simulink model "vertical_smm_with_lqr_3d"  (R2014b)
settings: Solver=FixedStepDiscrete  StartTime=0.0  StopTime=inf  FixedStep=sample_time  RelTol=1e-3
values from neighbouring files (symbols this model uses):
  forward_dx = [-0.304875592207 -0.274388032987 -0.243900473766 -0.213412914545 -0.182925355324 -0.152437796104 -0.121950236883 -0.0914626776622 -0.0609751184415 -0.0304875592207 0 0.0304875592207 ... (714 elements, 21x34)]    [ref_trajs.mat]
  forward_dx_of_dxstar = [-1.3048755994 -1.25487559904 -1.20487559868 -1.15487559832 -1.10487559796 -1.0548755976 -1.00487559724 -0.954875596883 -0.904875596523 -0.854875596164 -0.804875595804 -0.754875595707 ... (29274 elements, 41x21x34)]    [ref_trajs.mat]
  forward_x = [0.0961104217981 0.0864993796183 0.0768883374385 0.0672772952586 0.0576662530788 0.048055210899 0.0384441687192 0.0288331265394 0.0192220843596 0.00961104217981 0 -0.00961104217981 ... (714 elements, 21x34)]    [ref_trajs.mat]
  forward_x_of_dxstar = [0.247353819189 0.239791649319 0.232229479449 0.22466730958 0.21710513971 0.209542969841 0.201980799971 0.194418630102 0.186856460232 0.179294290363 0.171732120493 0.164169950675 ... (29274 elements, 41x21x34)]    [ref_trajs.mat]
  target_dx_range = [-1 -0.95 -0.9 -0.85 -0.8 -0.75 -0.7 -0.65 -0.6 -0.55 -0.5 -0.45 ... (41 elements, 1x41)]    [ref_trajs.mat]
undefined symbols (not defined in the file or in its folder): A_kalman_fourbar_gear, A_kalman_transverse, A_kalman_vertical, A_lpf_dtau, A_lpf_leg_spring, B1_lpf_dtau, B1_lpf_leg_spring, B2_lpf_dtau, B2_lpf_leg_spring, B_dx_versus_x0, B_kalman_fourbar_gear, B_kalman_transverse, B_kalman_vertical, backwards_K_front_of_t_row1, backwards_K_front_of_t_row2, backwards_K_sag_of_t, C_kalman_fourbar_gear, C_kalman_transverse, C_kalman_vertical, com_leg_motor, com_torso, contact_threshold, control_start_time, d_vertical_com, deadbeat_enabled, desired_com_forward_velocity, desired_com_lateral_velocity, desired_initial_leg_roll_left, desired_initial_leg_roll_right, desired_lateral_symmetry_angle, desired_torso_pitch, desired_torso_roll, Discrete, fcut_contact, forward_velocity_target_step, g, HIP_MTR_MAX_CONT_TORQUE, i_leg_motor, i_robot, i_torso, initial_dx_estimate, initial_dy_estimate, initial_dz_estimate, initial_z_estimate, j_motor, j_segments, K_left_lat_flight, K_left_lat_flight_winch, k_LQR_vertical, K_right_lat_flight, K_right_lat_flight_winch, k_sea, k_vertical_winch, kalman_load_to_deflect_transmission, kalman_stance_slip_threshold, kd_motor, kp_motor, l_retract_delta, l_retract_swing_max, l_retract_swing_min ... (+58)
libraries: simulink x8, ctrlSharedLib x7
(part 4 of 4)

== matlab function vertical_smm_with_lqr_3d/Control/Behavior Control/Primary Leg Behavior/Running/Stance/COM X,Y,Z  trajectory generation ==
  data: enable_hopping input; x_0 output size=1; y_0 output size=1; z_ref output size=1; dz_ref output size=1; ddz_ref output size=1; x_ref output size=1; dx_ref output size=1; y_ref output size=1; dy_ref output size=1; t input size=1; dx0 input; dy0 input; target_DX input; target_DY input; z_rest_new parameter; z_amplitude parameter; spring_frequency parameter; phase_0 parameter; forward_x_of_dxstar parameter; forward_dx_of_dxstar parameter; forward_x parameter; forward_dx parameter; target_dx_range parameter; T_s parameter
%% COM trajectory generation for stance & foot placement for flight

% Outputs:
% x_0: desired x position for foot at touchdown
% y_0: desired y position for foot at touchdown
% [z_ref, dz_ref, ddz_ref]: reference trajectory for vertical
% [x_ref, dx_ref]: reference trajectory for forward
% [y_ref, dy_ref]: reference trajectory for lateral

% Inputs:
% t: time since touchdown
% dx0: touchdown x velocity
% dy0: touchdown y velocity
% target_DX: desired x velocity at takeoff
% s_duration: nominal stance time
% z_rest_new: z height of oscillation
% target_dx_range: full range of possible x velocities in lookup table
% forward_x_of_dxstar: master lookup table for x trajectories
% T_s: tabled vector from 0 to s_duration

function [x_0, y_0,...
          z_ref, dz_ref, ddz_ref, ...
          x_ref, dx_ref, y_ref, dy_ref] ...
          = ReferenceTrajectory(enable_hopping, t, dx0, dy0, target_DX, target_DY, z_rest_new, z_amplitude, ...
            spring_frequency, phase_0, forward_x_of_dxstar, forward_dx_of_dxstar, ...
            forward_x, forward_dx, target_dx_range, T_s)
        
  % Z trajectory during stance
    if enable_hopping
        z_ref =  z_rest_new + z_amplitude*sin(spring_frequency*t+phase_0);
        dz_ref = z_amplitude*spring_frequency*cos(spring_frequency*t+phase_0);
        ddz_ref = -z_amplitude*spring_frequency^2*sin(spring_frequency*t+phase_0);
    else
        z_ref = z_rest_new - z_amplitude;
        dz_ref = 0;
        ddz_ref = 0;
    end
    
  % [X, dX] trajectory from 0 to s_duration
  forward_x_given_dxstar = squeeze(interp1(target_dx_range, forward_x_of_dxstar, target_DX));
  forward_dx_given_dxstar = squeeze(interp1(target_dx_range, forward_dx_of_dxstar, target_DX));
    
  % saturate t and initial velocity to reference library
  t_sat = max( min(t, T_s(end)), 0);
  dx0 = max( min(dx0, max(forward_dx_given_dxstar(:,1))), min(forward_dx_given_dxstar(:,1)) );
  x_ref  = interp2(T_s, forward_dx_given_dxstar(:,1), forward_x_given_dxstar, t_sat, dx0);
  dx_ref = interp2(T_s, forward_dx_given_dxstar(:,1), forward_dx_given_dxstar, t_sat, dx0);
  x_0 = interp1(forward_dx_given_dxstar(:,1), forward_x_given_dxstar(:,1), dx0);

  % for now, keep dy_star = 0;
  dy0 = max( min(dy0, max(forward_dx(:,1))), min(forward_dx(:,1)) );
  y_ref =  interp2(T_s, forward_dx(:,1), forward_x, t_sat, dy0);
  dy_ref = interp2(T_s, forward_dx(:,1), forward_dx, t_sat, dy0);
  y_0 = interp1(forward_dx(:,1), forward_x(:,1), dy0);
end

== matlab function vertical_smm_with_lqr_3d/Control/Behavior Control/Primary Leg Behavior/Running/Stance/Lookup finite horizon LQR gain ==
  data: K_sag output; t_forward input; backwards_K_sag_of_t parameter; backwards_K_front_of_t_row1 parameter; backwards_K_front_of_t_row2 parameter; T_lqr parameter; stance_duration parameter; K_front output
%% Interpolates pregenerated finite horizon LQR gain tables 
% sagittal_state: [X, Pitch, dX, dPtich]
% frontal state: [Y; Roll; sym; dY; dRoll; angular_momentum];
function [K_sag, K_front]  =  FiniteHorizonLQRLookup(t_forward, backwards_K_sag_of_t, backwards_K_front_of_t_row1, backwards_K_front_of_t_row2, T_lqr, stance_duration)
  t = stance_duration - t_forward; % gains are scheduled w.r.t time until end.                                     
  t = min(max(t, min(T_lqr)), max(T_lqr));
  K_sag = interp1(T_lqr, backwards_K_sag_of_t, t);

  % inputs for frontal LQR: backwards_K_front_of_t_row1, backwards_K_front_of_t_row2
  K_front_row1 = interp1(T_lqr, backwards_K_front_of_t_row1, t);
  K_front_row2 = interp1(T_lqr, backwards_K_front_of_t_row2, t);
  K_front = [K_front_row1; K_front_row2];
end

== matlab function vertical_smm_with_lqr_3d/Control/Behavior Control/Primary Leg Behavior/Running/Flight/Convert Foot Position to Joint Angles + Leg Length  ==
  data: deadbeat input; desired_leg_length output; X_star input; Y_star input; Z_star input; right_left input; com_pelvis_body input; desired_alpha output; desired_beta output; dcom_pelvis_body input; roll input; pitch input; sagittal_angle input; lateral_angle input; leg_length input; lateral_offset parameter; max_leg_length parameter; desired_initial_leg_roll_right parameter; desired_initial_leg_roll_left parameter; z_land parameter; d_vertical_com parameter
function [ desired_leg_length, desired_alpha, desired_beta ]  =  ...
          ConvertToJointAnglesAndLegLength(deadbeat, X_star, Y_star, Z_star, right_left,...
                           com_pelvis_body, dcom_pelvis_body, ...
                           roll, pitch, sagittal_angle, lateral_angle, leg_length,...
                           lateral_offset, max_leg_length, desired_initial_leg_roll_right, desired_initial_leg_roll_left, z_land, d_vertical_com) 

    q = [roll(1), pitch(1), sagittal_angle(1), lateral_angle(1), leg_length(1)];
    dq = [roll(2), pitch(2), sagittal_angle(2), lateral_angle(2), leg_length(2)];
    [desired_alpha, desired_beta, desired_leg_length]  =  ConvertFootPositionToLegAnglesAndLegLength(X_star, Y_star, Z_star, right_left, com_pelvis_body, dcom_pelvis_body, q, dq, lateral_offset, max_leg_length);   
                       
    if ~deadbeat
        desired_leg_length = [z_land-d_vertical_com; 0; 0];
        desired_alpha = [pi; 0; 0];
        desired_beta = [desired_initial_leg_roll_left; 0; 0];
        if right_left
            desired_beta = [desired_initial_leg_roll_right; 0; 0];
        end
    end
    
end

== matlab function vertical_smm_with_lqr_3d/Control/Behavior Control/Primary Leg Behavior/Running/Circular Buffer/Buffer7 ==
  data: data input; buffer output size=recorded_steps; trigger input; buffer_size input
function buffer  = buffer_data(data, trigger, buffer_size)

    persistent buffer_memory
    coder.varsize('buffer_memory',100);
    if isempty(buffer_memory)
        buffer_memory = [];
    end
    
    if trigger
        buffer_memory = [data; buffer_memory];
        if size(buffer_memory, 1) > buffer_size
            buffer_memory = buffer_memory(1:buffer_size,:);
        end
    end
    
    buffer = buffer_memory;

end

== matlab function vertical_smm_with_lqr_3d/Control/Behavior Control/Secondary Leg Behavior/Virtual Leg to Four Bar ==
  data: l_leg input; dl_leg input; ddl_leg input; phi input; dphi input; ddphi input; back output; dback output; ddback output; front output; dfront output; ddfront output
function [back, dback, ddback, front, dfront, ddfront] = VirtualLegToFourBar(l_leg, dl_leg, ddl_leg, phi, dphi, ddphi)
    [back, dback, ddback, front, dfront, ddfront] = VirtualLegToFourBar(l_leg, dl_leg, ddl_leg, phi, dphi, ddphi);
end

== matlab function vertical_smm_with_lqr_3d/Control/Behavior Control/Primary Leg Behavior/Running/Closed Loop Compensation/CLOSED LOOP COMPENSATION X FOR VAIRABLE SPEED ==
  data: A_cl input; epsilon input; c input; delta_s_i input; dx_star input; B_cl input; delta_ux output
function delta_ux  = closed_loop_compensation_dxstar...
         (A_cl,epsilon, c, delta_s_i, dx_star, B_cl)
% assume form of delta_s_{i+1} = A_cl*delta_s_i + epsilon +c*dx_star + B_cl*delta_ux
% where delta measures deviation from deadbeat case. solve for
% delta_ux = (-A_cl*delta_s_i-epsilon - c*dxstar)/B_cl to achieve deadbeat
delta_ux = (-A_cl*delta_s_i - epsilon - c*dx_star)/B_cl;

== matlab function vertical_smm_with_lqr_3d/Control/Behavior Control/Primary Leg Behavior/Running/Closed Loop Compensation/ESTIMATE CLOSED LOOP ERROR X FOR VARIABLE SPEED ==
  data: dx_land_hist input; A_cl output; delta_ux_hist input; dx_lift_hist input; dx_star_hist input; B_dx_versus_x0 parameter; W_real input; epsilon_0 output; c output; A_cl_nb output; epsilon_0_nb output; c_nb output
function [A_cl, epsilon_0, c, ...
          A_cl_nb, epsilon_0_nb, c_nb] = error_fitting_dxstar...
         (dx_land_hist, delta_ux_hist, dx_lift_hist, dx_star_hist,...
          B_dx_versus_x0, W_real)
% data_length = min([length(dx_lift_hist), filter_length]);
data_length = length(dx_lift_hist);
assert(data_length < 100);
% add fake data
fake_dx_land_err_magnitude = 0.1; fake_dx_star_magnitude = 0.1;
[fgrid_dx_land_err, fgrid_dx_star, fgrid_dx_lift_err] = ...
    meshgrid(fake_dx_land_err_magnitude*[-1 1],fake_dx_star_magnitude*[-1 1],0);
fake_data_length = numel(fgrid_dx_land_err);
fake_dx_land_err = fgrid_dx_land_err(:);
fake_dx_star = fgrid_dx_star(:);
fake_dx_lift_err = fgrid_dx_lift_err(:);
fake_delta_ux = zeros(fake_data_length,1);
% assert(fake_data_length<100);
% assert(filter_length<100);
% fake_dx_land_err = linspace(-0.1, 0.1, fake_data_length)';
% fake_dx_lift_err = zeros(fake_data_length,1);
% fake_delta_ux = zeros(fake_data_length,1);
% fake_dx_star = linspace(-0.25, 0.25, fake_data_length)';
dx_land_err = [reshape(dx_land_hist(1:data_length)-dx_star_hist(1:data_length),...
                       data_length, 1); fake_dx_land_err];
dx_lift_err = [reshape(dx_lift_hist(1:data_length)-dx_star_hist(1:data_length),...
                       data_length, 1); fake_dx_lift_err];
dx_star = [reshape(dx_star_hist(1:data_length), data_length,1); fake_dx_star];
delta_ux = [reshape(delta_ux_hist(1:data_length), data_length, 1); fake_delta_ux];
% weighted least squares
W = diag([W_real*ones(1,data_length), ones(1,fake_data_length)]);
Y = dx_lift_err - B_dx_versus_x0*delta_ux;
X = [dx_land_err, dx_star, ones(data_length+fake_data_length,1)];
% linear regression for s_{i+1}-s0 = A_cl*(s_i-s0) + epsilon_0 + c(s0) + B*delta_u
% solve for Y = X*beta, beta column vector
beta_hat = (X'*W*X)\X'*W*Y;
W_nobias = diag([W_real*ones(1,data_length), 0.001*ones(1,fake_data_length)]);
beta_hat_nobias = (X'*W_nobias*X)\X'*W_nobias*Y;
A_cl = beta_hat(1);
c = beta_hat(2);
epsilon_0 = beta_hat(3);
A_cl_nb = beta_hat_nobias(1);
c_nb = beta_hat_nobias(2);
epsilon_0_nb = beta_hat_nobias(3);

== matlab function vertical_smm_with_lqr_3d/Control/Behavior Control/Primary Leg Behavior/Running/Closed Loop Compensation/CLOSED LOOP COMPENSATION Y FOR VAIRABLE SPEED ==
  data: A_cl input; epsilon input; c input; delta_s_i input; dx_star input; B_cl input; delta_ux output
function delta_ux  = closed_loop_compensation_dxstar...
         (A_cl,epsilon, c, delta_s_i, dx_star, B_cl)
% assume form of delta_s_{i+1} = A_cl*delta_s_i + epsilon +c*dx_star + B_cl*delta_ux
% where delta measures deviation from deadbeat case. solve for
% delta_ux = (-A_cl*delta_s_i-epsilon - c*dxstar)/B_cl to achieve deadbeat
delta_ux = (-A_cl*delta_s_i - epsilon - c*dx_star)/B_cl;

== matlab function vertical_smm_with_lqr_3d/Control/Behavior Control/Primary Secondary Leg Swap/ToggleRightLeftLeg ==
  data: toggle input boolean; right_left output double; previous_right_left input double
function right_left = ToggleRightLeftLeg(toggle, previous_right_left)
    
    if toggle
        right_left = -previous_right_left + 1;
    else
        right_left = previous_right_left;
    end

end

== matlab function vertical_smm_with_lqr_3d/Control/Behavior Control/Force Estimation/3D Forward Dynamics yawed ==
  data: right_or_left input; torso_roll input size=2; torso_pitch input double size=2; torso_yaw input double size=2; primary_sagittal_leg_angle input double size=2; primary_leg_length input double size=2; primary_leg_roll input double size=2; secondary_leg_roll input double size=2; primary_leg_torque input; primary_leg_force input; primary_lateral_torque input; secondary_lateral_torque input; R_GRF output double size=3; L_GRF output size=3; ddroll output double; g parameter; m_leg_motor parameter; m_torso parameter; i_torso parameter; i_leg_motor parameter; lateral_offset parameter; com_torso parameter
%% Forward 3D ATRIAS dynamics
function [R_GRF, L_GRF, ddroll]  =  ForwardDynamics3D(right_or_left, ...
                                                      torso_roll, torso_pitch, torso_yaw, ...
                                                      primary_sagittal_leg_angle, primary_leg_length,...
                                                      primary_leg_roll, secondary_leg_roll, ...
                                                      primary_leg_torque, primary_leg_force, ...
                                                      primary_lateral_torque, secondary_lateral_torque, ...
                                                      g, m_leg_motor, m_torso, i_torso, i_leg_motor, lateral_offset, com_torso)

    d = norm(com_torso(2:3));
    It = mean(i_torso);
    Im = mean(i_leg_motor);
    
    phi    = torso_roll(1);                    % roll
    theta  = torso_pitch(1);                   % pitch
    alpha1 = primary_sagittal_leg_angle(1);    % primary sagittal leg angle
    beta1  = primary_leg_roll(1);              % primary leg roll
    beta2  = secondary_leg_roll(1);            % secondary leg roll
    l1     = primary_leg_length(1);            % primary leg length
    
    dphi    = torso_roll(2);
    dtheta  = torso_pitch(2);
    dpsi    = torso_yaw(2);
    dalpha1 = primary_sagittal_leg_angle(2);
    dbeta1  = primary_leg_roll(2);
    dbeta2  = secondary_leg_roll(2);
    dl1     = primary_leg_length(2);
    
    
    tau_a1 = primary_leg_torque;
    tau_b1 = primary_lateral_torque;
    tau_b2 = secondary_lateral_torque;
    F_l1 = primary_leg_force;

    if right_or_left == 1
      A = A_fwd_yawed_right(lateral_offset,d,m_leg_motor,m_torso,It,Im,phi,theta,alpha1,beta1,beta2,l1);
      B = B_fwd_yawed_right(lateral_offset,d,g,m_leg_motor,m_torso,It,Im,phi,theta,alpha1,beta1,beta2,l1,dphi,dtheta,dpsi,dalpha1,dbeta1,dbeta2,dl1,tau_a1,tau_b1,tau_b2,F_l1);
    else
      A = A_fwd_yawed_left(lateral_offset,d,m_leg_motor,m_torso,It,Im,phi,theta,alpha1,beta1,beta2,l1);
      B = B_fwd_yawed_left(lateral_offset,d,g,m_leg_motor,m_torso,It,Im,phi,theta,alpha1,beta1,beta2,l1,dphi,dtheta,dpsi,dalpha1,dbeta1,dbeta2,dl1,tau_a1,tau_b1,tau_b2,F_l1);
    end
    
    x_fwd = A \ B;
    ddroll = x_fwd(4);
    GRF = zeros(3,1);
    GRF(1) = x_fwd(11);
    GRF(2) = x_fwd(12);
    GRF(3) = x_fwd(13); 
    
    if right_or_left == 1
        R_GRF = GRF;
        L_GRF = [0;0;0];
    else
        R_GRF = [0;0;0];
        L_GRF = GRF;
    end
end

== matlab function vertical_smm_with_lqr_3d/Control/Behavior Control/Primary Leg Behavior/Running/Flight/Avoid Hitting Mechanical Limits ==
  data: back_cmd output double; front_cmd output double; dback_cmd output double; dfront_cmd output double; ddback_cmd output double; ddfront_cmd output double; back_desired input; dback_desired input; ddback_desired input; front_desired input; dfront_desired input; ddfront_desired input; min_front_bar_angle parameter; max_front_bar_angle parameter; min_back_bar_angle parameter; max_back_bar_angle parameter
%% Avoid joint limits by ensuring we don't command velocities/accelerations that would push us into them when we are close to them.
function [back_cmd, front_cmd, dback_cmd, dfront_cmd, ddback_cmd, ddfront_cmd] ...
    = AvoidFourbarLimits(back_desired,dback_desired, ddback_desired, ...
          front_desired, dfront_desired, ddfront_desired, ...
          min_front_bar_angle, max_front_bar_angle, min_back_bar_angle, max_back_bar_angle)
    [back_cmd, front_cmd, dback_cmd, dfront_cmd, ddback_cmd, ddfront_cmd] = AvoidFourbarLimits(back_desired,dback_desired, ddback_desired, front_desired, dfront_desired, ddfront_desired, min_front_bar_angle, max_front_bar_angle, min_back_bar_angle, max_back_bar_angle);
end

== matlab function vertical_smm_with_lqr_3d/Control/Behavior Control/Primary Leg Behavior/Running/Flight/Virtual Leg to Four Bar ==
  data: l_leg input; dl_leg input; ddl_leg input; phi input; dphi input; ddphi input; back output; dback output; ddback output; front output; dfront output; ddfront output
function [back, dback, ddback, front, dfront, ddfront] = VirtualLegToFourBar(l_leg, dl_leg, ddl_leg, phi, dphi, ddphi)
    [back, dback, ddback, front, dfront, ddfront] = VirtualLegToFourBar(l_leg, dl_leg, ddl_leg, phi, dphi, ddphi);
end

== matlab function vertical_smm_with_lqr_3d/Control/Behavior Control/Primary Leg Behavior/Running/Flight/Lateral Flight Control ==
  data: hopping input; tau_primary output; tau_secondary output; RightLeftPrimary input; TorsoRoll input; LLegRoll input; RLegRoll input; Beta1_star input; Roll_star input; K_right_lat_flight parameter; K_left_lat_flight parameter; K_right_lat_flight_winch parameter; K_left_lat_flight_winch parameter; Q_phibeta1beta2 parameter; Q_phibeta1beta2_winch parameter; m_torso parameter; m_leg_motor parameter; com_torso parameter; i_torso parameter; i_leg_motor parameter; g parameter; lateral_offset parameter; adjusted_ref output; feedforward output; desired_initial_leg_roll_left parameter; desired_initial_leg_roll_right parameter
% full_state = [Roll; Beta1; Beta2; dRoll; dBeta1; dBeta2];
function [tau_primary, tau_secondary, ...
          adjusted_ref, feedforward] = lateral_flight_control(hopping, RightLeftPrimary,...
          TorsoRoll, LLegRoll, RLegRoll, Beta1_star, Roll_star,...
          K_right_lat_flight, K_left_lat_flight, K_right_lat_flight_winch, K_left_lat_flight_winch, Q_phibeta1beta2, Q_phibeta1beta2_winch,...
          m_torso, m_leg_motor, com_torso, i_torso, i_leg_motor, g, lateral_offset, desired_initial_leg_roll_left, desired_initial_leg_roll_right)

    d = norm(com_torso(2:3));
    It_f = i_torso(1);
    Im_f = i_leg_motor(1); 
    phidphi = TorsoRoll; 
    symdsym = LLegRoll-RLegRoll;
    ang_mom = phidphi(2)*(m_torso*d^2 + It_f + 2*(m_leg_motor*lateral_offset^2+ Im_f)) -symdsym(2)*(m_leg_motor*lateral_offset^2+Im_f);

    if RightLeftPrimary == 1
        Beta1 = RLegRoll;
        Beta2 = LLegRoll;
        Beta2_star = [desired_initial_leg_roll_left; 0; 0];
    else
        Beta1 = LLegRoll;
        Beta2 = RLegRoll;
        Beta2_star = [desired_initial_leg_roll_right; 0; 0];
    end    
    
    if ~hopping
        Q_phibeta1beta2 = Q_phibeta1beta2_winch;
        K_right_lat_flight = K_right_lat_flight_winch;
        K_left_lat_flight = K_left_lat_flight_winch;
    end

    ref_old = [Roll_star(1); Beta1_star(1); Beta2_star(1)];
    dref_old = [0; Beta1_star(2); Beta2_star(2)];
    ddref_old = [0; Beta1_star(3); Beta2_star(3)];
    
    % eliminate beta2 from state using momentum:
    % s_old = T*s_new+D(t); s_new = [phi; beta1];
    % dbeta_R = L/(Im_f+mm*r^2) - (It_f+mm*d^2+2*Im_f+2*mm*r^2)/(Im_f+mm*r^2)*dphi + dbeta_L 
    % beta_R = beta_R0 + L/(Im_f+mm*r^2)*t - ((It_f+mm*d^2+2*Im_f+2*mm*r^2)/(Im_f+mm*r^2)*(phi-phi0) + (beta_L-beta_L0)
    % beta_R = [beta_R0-b1*phi0-b2*beta_L0 + a*t + b1*phi + b2*beta_L;
    
    if RightLeftPrimary == 1 % beta_2 is beta_L, beta_1 is beta_R, eliminate beta2
      a = -ang_mom/(Im_f+m_leg_motor*lateral_offset^2);
      b1 = (It_f+m_torso*d^2+2*Im_f+2*m_leg_motor*lateral_offset^2)/(Im_f+m_leg_motor*lateral_offset^2); b2 = 1;
    else
      a = +ang_mom/(Im_f+m_leg_motor*lateral_offset^2);
      b1 = -(It_f+m_torso*d^2+2*Im_f+2*m_leg_motor*lateral_offset^2)/(Im_f+m_leg_motor*lateral_offset^2); b2 = 1;
    end
    
    T = [eye(2); b1, b2];
    %  D = [0; 0; 0; 0; beta_R0 - b1*phi0 - b2*beta_L0 + a*t; a];
    D = [0;0; Beta2(1) - b1*phidphi(1) - b2*Beta1(1)];
    
    % old cost (state s)  (s-s_ref)' * Q *(s-s_ref);
    % new cost (state r) =(T*r+D-s_ref)'*Q*(T*r+D-s_ref);
    %                    =(r+ (T'QT)^{-1}T'Q(D-s_ref))'*T'QT*
    %                     (r + (T'QT)^{-1}T'Q(D-s_ref))
    
    
    Q_new = T'*Q_phibeta1beta2*T;
    ref_new = Q_new\T'*Q_phibeta1beta2*(ref_old-D);
    ref_new_vel = Q_new\T'*Q_phibeta1beta2*(dref_old - [0;0; a]);
    ref_accels = Q_new\T'*Q_phibeta1beta2*(ddref_old);

    % A_phidphi_betadbeta1 = [0 1 0 0; 0 0 0 0; 0 0 0 1; 0 0 0 0];
    % assume beta1 is right
    if RightLeftPrimary == 1
        B_new_state = [0 0; 0 0; -1/(It_f+m_torso*d^2), 1/(It_f+m_torso*d^2); 1/(It_f+m_torso*d^2)+1/(Im_f+m_leg_motor*lateral_offset^2), -1/(It_f+m_torso*d^2)];
    else
        B_new_state = [0 0; 0 0; 1/(It_f+m_torso*d^2), -1/(It_f+m_torso*d^2); 1/(It_f+m_torso*d^2)+1/(Im_f+m_leg_motor*lateral_offset^2), -1/(It_f+m_torso*d^2)];
    end      
    
    %   K = lqr(A_phidphi_betadbeta1, B_phidphi_betadbeta1, Q_new, R_lat_flight);
    if RightLeftPrimary == 1
      K = K_right_lat_flight;
    else
      K = K_left_lat_flight;
    end

    new_state = [phidphi(1); Beta1(1); phidphi(2); Beta1(2)];
    new_ref_traj = [ref_new; ref_new_vel];

    feedforward = B_new_state([3 4],:)\ref_accels;
    if ~hopping, feedforward = -(m_leg_motor)*g*lateral_offset*ones(2,1); end
    tau_lqr = feedforward - K*(new_state-new_ref_traj);
    tau_1 = tau_lqr(1); tau_2 = tau_lqr(2);
    implied_beta2_star = [0 0 1]*(T*ref_new+D);
    implied_dbeta2_star = [0 0 1]*(T*ref_new_vel+[0; 0; a]);
    % implied_betadbeta2_star = [0 0 0 0 1 0; 0 0 0 0 0 1]*(T*ref_new+D);
    adjusted_ref = [ref_new; implied_beta2_star; ref_new_vel; implied_dbeta2_star];

    tau_primary = tau_1;
    tau_secondary = tau_2;

== matlab function vertical_smm_with_lqr_3d/Control/Behavior Control/Secondary Leg Behavior/Mirrored Leg Length Target ==
  data: primary_l_leg input; l_leg output; dl_leg output; primary_dl_leg input; l_retract_swing_min parameter; l_retract_swing_max parameter; ddl_leg output; l_retract_delta parameter
function [l_leg, dl_leg, ddl_leg] = LegLengthTarget(primary_l_leg, primary_dl_leg, l_retract_swing_min, l_retract_swing_max, l_retract_delta)

    l_leg = primary_l_leg - l_retract_delta;
    dl_leg = 0;
    ddl_leg = 0;
    if l_leg > l_retract_swing_min && l_leg < l_retract_swing_max
        dl_leg = primary_dl_leg;
    else
        l_leg = max(min(l_leg, l_retract_swing_max), l_retract_swing_min);
    end

end

== matlab function vertical_smm_with_lqr_3d/Fourbar Gearside Kalman Filter/External Trunk Torque Estimate ==
  data: grf_xz input; rotor_torque input; spring_torque input; tau_trunk output; torso_pitch input; d_vertical_com parameter; LEG_MTR_GEAR_RATIO parameter
function tau_trunk = tau_trunk(grf_xz, rotor_torque, spring_torque, torso_pitch, d_vertical_com, LEG_MTR_GEAR_RATIO )
    d = d_vertical_com;
    theta = torso_pitch;
    N = LEG_MTR_GEAR_RATIO;
    tau_trunk = sum(-rotor_torque + -(N-1)/N*spring_torque) + (-d*cos(theta)*grf_xz(1) + d*sin(theta)*grf_xz(2));
end

== matlab function vertical_smm_with_lqr_3d/Fourbar Gearside Kalman Filter/Covariance Estimates ==
  data: spring_torque input; absolute_gear input; current_position_estimate input; state_uncertainty input; Q1 output; R1 output; Q2 output; R2 output; R_kalman_absolute_normal parameter; R_kalman_absolute_fail parameter; R_kalman_incremental_unloaded parameter; R_kalman_incremental_loaded parameter; kalman_load_to_deflect_transmission parameter; Q3 output; R3 output; Q4 output; R4 output; max_absolute_measurement_innovation parameter; k_sea parameter; Q_kalman_spring_torque parameter; Q_kalman_rotor_torque parameter; Q_kalman_trunk_torque parameter; sample_time parameter
function [Q1, R1, Q2, R2, Q3, R3, Q4, R4] = covariance( spring_torque, absolute_gear, current_position_estimate, state_uncertainty, R_kalman_absolute_normal, R_kalman_absolute_fail, R_kalman_incremental_unloaded, R_kalman_incremental_loaded, kalman_load_to_deflect_transmission, max_absolute_measurement_innovation, k_sea, Q_kalman_spring_torque, Q_kalman_rotor_torque, Q_kalman_trunk_torque, sample_time)

    persistent previous_absolute_gear
    if isempty(previous_absolute_gear)
        previous_absolute_gear = absolute_gear;
    end
    
    % Measurement covariance
    R_absolute = ones(4,1)*R_kalman_absolute_normal;
    dropped_out = previous_absolute_gear == absolute_gear;
    out_of_range = abs(current_position_estimate - absolute_gear) > max_absolute_measurement_innovation;
    R_absolute(dropped_out | out_of_range) = R_kalman_absolute_fail;
    
    R_incremental_scale = min(abs(spring_torque)/kalman_load_to_deflect_transmission, 1);
    R_incremental = R_incremental_scale*R_kalman_incremental_loaded + (1-R_incremental_scale)*R_kalman_incremental_unloaded;
    
    R1 = diag([R_absolute(1), R_incremental(1)])/sample_time;
    R2 = diag([R_absolute(2), R_incremental(2)])/sample_time;
    R3 = diag([R_absolute(3), R_incremental(3)])/sample_time;
    R4 = diag([R_absolute(4), R_incremental(4)])/sample_time;
    
    % Process noise covariance
    Q_spring_torque = k_sea'.^2.*(state_uncertainty + R_kalman_absolute_normal) + Q_kalman_spring_torque;

    Q1 = diag([Q_spring_torque(1), Q_kalman_rotor_torque, Q_kalman_trunk_torque]);
    Q2 = diag([Q_spring_torque(2), Q_kalman_rotor_torque, Q_kalman_trunk_torque]);
    Q3 = diag([Q_spring_torque(3), Q_kalman_rotor_torque, Q_kalman_trunk_torque]);
    Q4 = diag([Q_spring_torque(4), Q_kalman_rotor_torque, Q_kalman_trunk_torque]);

    previous_absolute_gear = absolute_gear;
end

== matlab function vertical_smm_with_lqr_3d/Fourbar Gearside Kalman Filter/eigen values 1 ==
  data: Z input; E output
function E = eigen(Z)
    E = real(eig(Z));
    E = sort(E);
end

== matlab function vertical_smm_with_lqr_3d/Fourbar Gearside Kalman Filter/eigen values 2 ==
  data: Z input; E output
function E = eigen(Z)
    E = real(eig(Z));
    E = sort(E);
end

== matlab function vertical_smm_with_lqr_3d/Fourbar Gearside Kalman Filter/eigen values 3 ==
  data: Z input; E output
function E = eigen(Z)
    E = real(eig(Z));
    E = sort(E);
end

== matlab function vertical_smm_with_lqr_3d/Fourbar Gearside Kalman Filter/eigen values4  ==
  data: Z input; E output
function E = eigen(Z)
    E = real(eig(Z));
    E = sort(E);
end

== matlab function vertical_smm_with_lqr_3d/Control/Behavior Control/Primary Leg Behavior/Running/Stance/3D Inverse Dynamics yawed ==
  data: right_or_left input; primary_leg_torque output double size=1; torso_roll input double size=2; torso_pitch input double size=2; torso_yaw input size=2; primary_sagittal_leg_angle input size=2; primary_leg_length input size=2; primary_leg_roll input size=2; secondary_leg_roll input size=2; GRF_desired input double size=3; ddRoll_desired input double size=1; g parameter; primary_lateral_torque output double size=1; secondary_lateral_torque output double size=1; primary_leg_force output double size=1; m_leg_motor parameter; m_torso parameter; i_torso parameter; i_leg_motor parameter; lateral_offset parameter; com_torso parameter
%% Inverse dynamics
function [primary_leg_torque, primary_lateral_torque, secondary_lateral_torque, primary_leg_force]  =  InverseDynamics3D(right_or_left,...
                                                                                                                         torso_roll, torso_pitch, torso_yaw, ...
                                                                                                                         primary_sagittal_leg_angle, primary_leg_length, ...
                                                                                                                         primary_leg_roll, secondary_leg_roll, ...
                                                                                                                         GRF_desired, ddRoll_desired, ...
                                                                                                                         g, m_leg_motor, m_torso, i_torso, i_leg_motor, lateral_offset, com_torso)

    d = norm(com_torso(2:3));
    It = mean(i_torso);
    Im = mean(i_leg_motor);
    
    phi    = torso_roll(1);                    % roll
    theta  = torso_pitch(1);                   % pitch
    alpha1 = primary_sagittal_leg_angle(1);    % primary sagittal leg angle
    beta1  = primary_leg_roll(1);              % primary leg roll
    beta2  = secondary_leg_roll(1);            % secondary leg roll
    l1     = primary_leg_length(1);            % primary leg length
    
    dphi    = torso_roll(2);
    dtheta  = torso_pitch(2);
    dpsi    = torso_yaw(2);
    dalpha1 = primary_sagittal_leg_angle(2);
    dbeta1  = primary_leg_roll(2);
    dbeta2  = secondary_leg_roll(2);
    dl1     = primary_leg_length(2);

    Fx = GRF_desired(1);
    Fy = GRF_desired(2);
    Fz = GRF_desired(3);
    ddphi = ddRoll_desired;

    if right_or_left == 1
      A = A_id_roll_yawed_right(lateral_offset,d,m_leg_motor,m_torso,It,Im,phi,theta,alpha1,beta1,beta2,l1);     
      B = B_id_roll_yawed_right(lateral_offset,d,g,m_leg_motor,m_torso,It,Im,phi,theta,alpha1,beta1,beta2,l1,dphi,dtheta,dpsi,dalpha1,dbeta1,dbeta2,dl1,Fx,Fy,Fz,ddphi);
    else
      A = A_id_roll_yawed_left(lateral_offset,d,m_leg_motor,m_torso,It,Im,phi,theta,alpha1,beta1,beta2,l1);     
      B = B_id_roll_yawed_left(lateral_offset,d,g,m_leg_motor,m_torso,It,Im,phi,theta,alpha1,beta1,beta2,l1,dphi,dtheta,dpsi,dalpha1,dbeta1,dbeta2,dl1,Fx,Fy,Fz,ddphi);
    end        
    x_id_roll = A \ B;
    primary_leg_torque = x_id_roll(10);
    primary_lateral_torque = x_id_roll(11);
    secondary_lateral_torque = x_id_roll(12);
    primary_leg_force = x_id_roll(13);
end

== matlab function vertical_smm_with_lqr_3d/Control/Behavior Control/Primary Leg Behavior/Running/Flight/Avoid Virtual Leg Length Limits ==
  data: l_leg_desired input; dl_leg_desired input; ddl_leg_desired input; l_leg_cmd output double; dl_leg_cmd output double; ddl_leg_cmd output double; min_leg_length parameter; max_leg_length parameter
%% Avoid virtual leg length limits by ensuring we don't command position/velocities/accelerations that would hit them.
function [l_leg_cmd, dl_leg_cmd, ddl_leg_cmd] = AvoidVirtualLengthLimits(l_leg_desired, dl_leg_desired, ddl_leg_desired, min_leg_length, max_leg_length)
    [l_leg_cmd, dl_leg_cmd, ddl_leg_cmd] = AvoidVirtualLengthLimits(l_leg_desired, dl_leg_desired, ddl_leg_desired, min_leg_length, max_leg_length);
end

== matlab function vertical_smm_with_lqr_3d/Control/Behavior Control/Primary Leg Behavior/Running/Flight/Calculate Time Until Touchdown ==
  data: z_dz input; t output; z_land parameter; g parameter
function t = EstimateTouchdown(z_dz, z_land, g)
  z_hat = z_dz(1); 
  dz_hat = z_dz(2);
  t = (-dz_hat-sqrt( max(dz_hat^2 - 4*g/2*(z_land-z_hat),0) ))/(-g);
end

== matlab function vertical_smm_with_lqr_3d/Control/Behavior Control/Primary Leg Behavior/Running/Closed Loop Compensation/ESTIMATE CLOSED LOOP ERROR Y FOR VARIABLE SPEED ==
  data: dx_land_hist input; A_cl output; delta_ux_hist input; dx_lift_hist input; dx_star_hist input; B_dx_versus_x0 parameter; W_real input; epsilon_0 output; c output; A_cl_nb output; epsilon_0_nb output; c_nb output
function [A_cl, epsilon_0, c, ...
          A_cl_nb, epsilon_0_nb, c_nb] = error_fitting_dxstar...
         (dx_land_hist, delta_ux_hist, dx_lift_hist, dx_star_hist,...
          B_dx_versus_x0, W_real)
% data_length = min([length(dx_lift_hist), filter_length]);
data_length = length(dx_lift_hist);
assert(data_length < 100);
% add fake data
fake_dx_land_err_magnitude = 0.1; fake_dx_star_magnitude = 0.1;
[fgrid_dx_land_err, fgrid_dx_star, fgrid_dx_lift_err] = ...
    meshgrid(fake_dx_land_err_magnitude*[-1 1],fake_dx_star_magnitude*[-1 1],0);
fake_data_length = numel(fgrid_dx_land_err);
fake_dx_land_err = fgrid_dx_land_err(:);
fake_dx_star = fgrid_dx_star(:);
fake_dx_lift_err = fgrid_dx_lift_err(:);
fake_delta_ux = zeros(fake_data_length,1);
% assert(fake_data_length<100);
% assert(filter_length<100);
% fake_dx_land_err = linspace(-0.1, 0.1, fake_data_length)';
% fake_dx_lift_err = zeros(fake_data_length,1);
% fake_delta_ux = zeros(fake_data_length,1);
% fake_dx_star = linspace(-0.25, 0.25, fake_data_length)';
dx_land_err = [reshape(dx_land_hist(1:data_length)-dx_star_hist(1:data_length),...
                       data_length, 1); fake_dx_land_err];
dx_lift_err = [reshape(dx_lift_hist(1:data_length)-dx_star_hist(1:data_length),...
                       data_length, 1); fake_dx_lift_err];
dx_star = [reshape(dx_star_hist(1:data_length), data_length,1); fake_dx_star];
delta_ux = [reshape(delta_ux_hist(1:data_length), data_length, 1); fake_delta_ux];
% weighted least squares
W = diag([W_real*ones(1,data_length), ones(1,fake_data_length)]);
Y = dx_lift_err - B_dx_versus_x0*delta_ux;
X = [dx_land_err, dx_star, ones(data_length+fake_data_length,1)];
% linear regression for s_{i+1}-s0 = A_cl*(s_i-s0) + epsilon_0 + c(s0) + B*delta_u
% solve for Y = X*beta, beta column vector
beta_hat = (X'*W*X)\X'*W*Y;
W_nobias = diag([W_real*ones(1,data_length), 0.001*ones(1,fake_data_length)]);
beta_hat_nobias = (X'*W_nobias*X)\X'*W_nobias*Y;
A_cl = beta_hat(1);
c = beta_hat(2);
epsilon_0 = beta_hat(3);
A_cl_nb = beta_hat_nobias(1);
c_nb = beta_hat_nobias(2);
epsilon_0_nb = beta_hat_nobias(3);

== matlab function vertical_smm_with_lqr_3d/Control/Behavior Control/Primary Leg Behavior/Running/Circular Buffer/Buffer ==
  data: data input; buffer output size=recorded_steps; trigger input; buffer_size input
function buffer  = buffer_data(data, trigger, buffer_size)

    persistent buffer_memory
    coder.varsize('buffer_memory',100);
    if isempty(buffer_memory)
        buffer_memory = [];
    end
    
    if trigger
        buffer_memory = [data; buffer_memory];
        if size(buffer_memory, 1) > buffer_size
            buffer_memory = buffer_memory(1:buffer_size,:);
        end
    end
    
    buffer = buffer_memory;

end

== matlab function vertical_smm_with_lqr_3d/Control/Behavior Control/Primary Leg Behavior/Running/Circular Buffer/Buffer1 ==
  data: data input; buffer output size=recorded_steps; trigger input; buffer_size input
function buffer  = buffer_data(data, trigger, buffer_size)

    persistent buffer_memory
    coder.varsize('buffer_memory',100);
    if isempty(buffer_memory)
        buffer_memory = [];
    end
    
    if trigger
        buffer_memory = [data; buffer_memory];
        if size(buffer_memory, 1) > buffer_size
            buffer_memory = buffer_memory(1:buffer_size,:);
        end
    end
    
    buffer = buffer_memory;

end

== matlab function vertical_smm_with_lqr_3d/Control/Behavior Control/Primary Leg Behavior/Running/Circular Buffer/Buffer2 ==
  data: data input; buffer output size=recorded_steps; trigger input; buffer_size input
function buffer  = buffer_data(data, trigger, buffer_size)

    persistent buffer_memory
    coder.varsize('buffer_memory',100);
    if isempty(buffer_memory)
        buffer_memory = [];
    end
    
    if trigger
        buffer_memory = [data; buffer_memory];
        if size(buffer_memory, 1) > buffer_size
            buffer_memory = buffer_memory(1:buffer_size,:);
        end
    end
    
    buffer = buffer_memory;

end

== matlab function vertical_smm_with_lqr_3d/Control/Behavior Control/Primary Leg Behavior/Running/Circular Buffer/Buffer3 ==
  data: data input; buffer output size=recorded_steps; trigger input; buffer_size input
function buffer  = buffer_data(data, trigger, buffer_size)

    persistent buffer_memory
    coder.varsize('buffer_memory',100);
    if isempty(buffer_memory)
        buffer_memory = [];
    end
    
    if trigger
        buffer_memory = [data; buffer_memory];
        if size(buffer_memory, 1) > buffer_size
            buffer_memory = buffer_memory(1:buffer_size,:);
        end
    end
    
    buffer = buffer_memory;

end

== matlab function vertical_smm_with_lqr_3d/Control/Behavior Control/Primary Leg Behavior/Running/Circular Buffer/Buffer4 ==
  data: data input; buffer output size=recorded_steps; trigger input; buffer_size input
function buffer  = buffer_data(data, trigger, buffer_size)

    persistent buffer_memory
    coder.varsize('buffer_memory',100);
    if isempty(buffer_memory)
        buffer_memory = [];
    end
    
    if trigger
        buffer_memory = [data; buffer_memory];
        if size(buffer_memory, 1) > buffer_size
            buffer_memory = buffer_memory(1:buffer_size,:);
        end
    end
    
    buffer = buffer_memory;

end

== matlab function vertical_smm_with_lqr_3d/Control/Behavior Control/Primary Leg Behavior/Running/Circular Buffer/Buffer5 ==
  data: data input; buffer output size=recorded_steps; trigger input; buffer_size input
function buffer  = buffer_data(data, trigger, buffer_size)

    persistent buffer_memory
    coder.varsize('buffer_memory',100);
    if isempty(buffer_memory)
        buffer_memory = [];
    end
    
    if trigger
        buffer_memory = [data; buffer_memory];
        if size(buffer_memory, 1) > buffer_size
            buffer_memory = buffer_memory(1:buffer_size,:);
        end
    end
    
    buffer = buffer_memory;

end

== matlab function vertical_smm_with_lqr_3d/Control/Behavior Control/State Estimation/Kalman Filtering/Measurement Noise Covariance Matricies ==
  data: R_transverse output; vertical_GRF_L input; vertical_GRF_R input; R_kalman_foot_stance parameter; R_kalman_foot_slip parameter; R_kalman_dfoot_stance parameter; R_kalman_dfoot_slip parameter; sample_time parameter; m_total_real parameter; g parameter; R_vertical output; kalman_stance_slip_threshold parameter
function [R_transverse, R_vertical] =...
         MeasurementNoiseCovariance(vertical_GRF_L, vertical_GRF_R, ...
           R_kalman_foot_stance, R_kalman_foot_slip, R_kalman_dfoot_stance, R_kalman_dfoot_slip, sample_time, m_total_real, g, kalman_stance_slip_threshold)

    % filter states: [dx_w]; [dy_w]; [dz_w];
    % measurements:  [dx_w-dfL + dfL_hat; dx_w-dfR + dfR_hat]; 

    ratio_L = max(0, min(vertical_GRF_L/(kalman_stance_slip_threshold*m_total_real*g),1)); % ratio is 0 if no load, 1 if at least equilibrium
    ratio_R = max(0, min(vertical_GRF_R/(kalman_stance_slip_threshold*m_total_real*g),1));
    R_transverse = diag([ratio_L*R_kalman_dfoot_stance + (1-ratio_L)*R_kalman_dfoot_slip, ...
                         ratio_R*R_kalman_dfoot_stance + (1-ratio_R)*R_kalman_dfoot_slip])/sample_time;
    R_vertical = diag([ratio_L*R_kalman_foot_stance  + (1-ratio_L)*R_kalman_foot_slip,...
                       ratio_L*R_kalman_dfoot_stance + (1-ratio_L)*R_kalman_dfoot_slip,...
                       ratio_R*R_kalman_foot_stance  + (1-ratio_R)*R_kalman_foot_slip,...
                       ratio_R*R_kalman_dfoot_stance + (1-ratio_R)*R_kalman_dfoot_slip])/sample_time;
end
